simulink model "inverseDynamicsTest"  (Simulink 7.7)
settings: Solver=FixedStepDiscrete  StartTime=0.0  StopTime=1000  FixedStep=0.01  RelTol=1e-3
libraries: WBCLibrary x7, utility x1
settings Model: Creator=iron  LastModifiedBy=iron

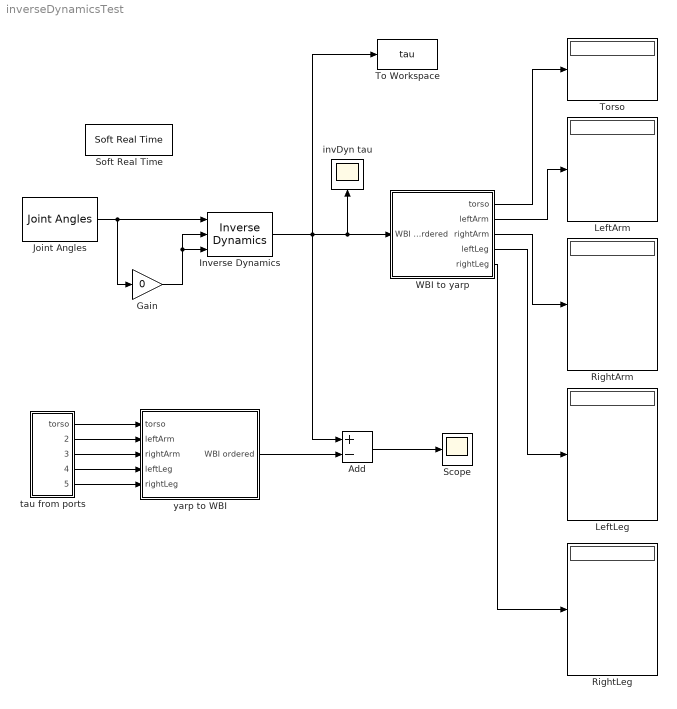
== system inverseDynamicsTest ==
  Add : Sum  Inputs=+-
  Gain : Gain  Gain=0
  Inverse Dynamics : WBCLibrary/wholeBodyModel/Dynamics/Inverse Dynamics  SystemSampleTime=-1  robotName=robotName  localName=localName
  Joint Angles : WBCLibrary/wholeBodyStates/Joint Angles  SystemSampleTime=-1  robotName=robotName  localName=localName
  LeftArm : Display
  LeftLeg : Display
  RightArm : Display
  RightLeg : Display
  Scope : Scope
      settings: YMin=-1.75  YMax=2.5
  Soft Real Time : utility/Soft Real Time  x=0.01
  To Workspace : ToWorkspace  VariableName=tau  SampleTime=-1  SaveFormat=Structure
  Torso : Display
  WBI to yarp : Subsystem
  invDyn tau : Scope
      settings: YMax=1.5
  tau from ports : Subsystem
  yarp to WBI : Subsystem
  wires:
  Joint Angles/1 -> Gain/1, Inverse Dynamics/1
  Gain/1 -> Inverse Dynamics/2, Inverse Dynamics/3
  Inverse Dynamics/1 -> To Workspace/1, Add/1, WBI to yarp/1(WBI ordered), invDyn tau/1
  Add/1 -> Scope/1
  yarp to WBI/1(WBI ordered) -> Add/2
  WBI to yarp/1(torso) -> Torso/1
  WBI to yarp/2(leftArm) -> LeftArm/1
  WBI to yarp/3(rightArm) -> RightArm/1
  WBI to yarp/4(leftLeg) -> LeftLeg/1
  WBI to yarp/5(rightLeg) -> RightLeg/1
  tau from ports/2(leftArm) -> yarp to WBI/2(leftArm)
  tau from ports/1(torso) -> yarp to WBI/1(torso)
  tau from ports/5(rightLeg) -> yarp to WBI/5(rightLeg)
  tau from ports/3(rightArm) -> yarp to WBI/3(rightArm)
  tau from ports/4(leftLeg) -> yarp to WBI/4(leftLeg)

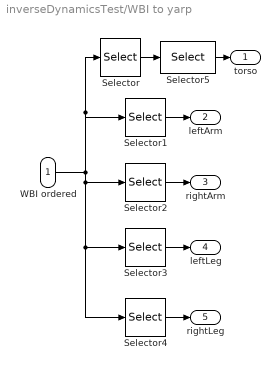
== system inverseDynamicsTest/WBI to yarp ==
  WBI ordered : Inport
  Selector : Selector  InputPortWidth=25  IndexOptions=Index vector (dialog)  Indices=[1 2 3]  OutputSizes=1
  Selector1 : Selector  InputPortWidth=25  IndexOptions=Index vector (dialog)  Indices=[4 5 6 7 8]  OutputSizes=1
  Selector2 : Selector  InputPortWidth=25  IndexOptions=Index vector (dialog)  Indices=[9 10 11 12 13]  OutputSizes=1
  Selector3 : Selector  InputPortWidth=25  IndexOptions=Index vector (dialog)  Indices=[14 15 16 17 18 19]  OutputSizes=1
  Selector4 : Selector  InputPortWidth=25  IndexOptions=Index vector (dialog)  Indices=[20 21 22 23 24 25]  OutputSizes=1
  Selector5 : Selector  InputPortWidth=3  IndexOptions=Index vector (dialog)  Indices=[3 2 1]  OutputSizes=1
  torso : Outport
  leftArm : Outport  Port=2
  rightArm : Outport  Port=3
  leftLeg : Outport  Port=4
  rightLeg : Outport  Port=5
  wires:
  Selector1/1 -> leftArm/1
  Selector2/1 -> rightArm/1
  Selector3/1 -> leftLeg/1
  Selector4/1 -> rightLeg/1
  WBI ordered/1 -> Selector/1, Selector1/1, Selector2/1, Selector4/1, Selector3/1
  Selector/1 -> Selector5/1
  Selector5/1 -> torso/1

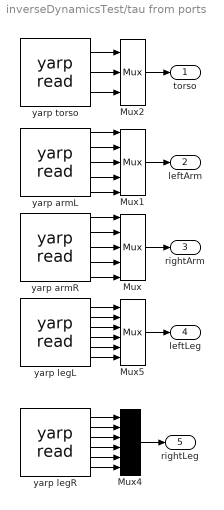
== system inverseDynamicsTest/tau from ports ==
  Mux : Mux  Inputs=5
  Mux1 : Mux  Inputs=5
  Mux2 : Mux  Inputs=3
  Mux4 : Mux  Inputs=6
  Mux5 : Mux  Inputs=6
  yarp armL : WBCLibrary/Utilities/yarp read  from='/icubGazeboSim/left_arm/analog:o/torques'  to='/tmp2:i'  num=5
  yarp armR : WBCLibrary/Utilities/yarp read  from='/icubGazeboSim/right_arm/analog:o/torques'  to='/tmp3:i'  num=5
  yarp legL : WBCLibrary/Utilities/yarp read  from='/icubGazeboSim/left_leg/analog:o/torques'  to='/tmp4:i'  num=6
  yarp legR : WBCLibrary/Utilities/yarp read  from='/icubGazeboSim/right_leg/analog:o/torques'  to='/tmp5:i'  num=6
  yarp torso : WBCLibrary/Utilities/yarp read  from='/icubGazeboSim/torso/analog:o/torques'  to='/tmp1:i'  num=3
  torso : Outport
  leftArm : Outport  Port=2
  rightArm : Outport  Port=3
  leftLeg : Outport  Port=4
  rightLeg : Outport  Port=5
  wires:
  yarp armR/1 -> Mux/1
  yarp armR/2 -> Mux/2
  yarp armR/3 -> Mux/3
  yarp armR/4 -> Mux/4
  yarp armR/5 -> Mux/5
  yarp armL/1 -> Mux1/1
  yarp armL/2 -> Mux1/2
  yarp armL/3 -> Mux1/3
  yarp armL/4 -> Mux1/4
  yarp armL/5 -> Mux1/5
  yarp torso/1 -> Mux2/1
  yarp torso/2 -> Mux2/2
  yarp torso/3 -> Mux2/3
  yarp legL/1 -> Mux5/1
  yarp legL/2 -> Mux5/2
  yarp legL/3 -> Mux5/3
  yarp legL/4 -> Mux5/4
  yarp legL/5 -> Mux5/5
  yarp legL/6 -> Mux5/6
  yarp legR/1 -> Mux4/1
  yarp legR/2 -> Mux4/2
  yarp legR/3 -> Mux4/3
  yarp legR/4 -> Mux4/4
  yarp legR/5 -> Mux4/5
  yarp legR/6 -> Mux4/6
  Mux2/1 -> torso/1
  Mux1/1 -> leftArm/1
  Mux/1 -> rightArm/1
  Mux5/1 -> leftLeg/1
  Mux4/1 -> rightLeg/1

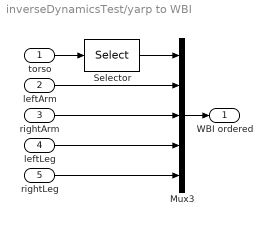
== system inverseDynamicsTest/yarp to WBI ==
  torso : Inport
  leftArm : Inport  Port=2
  rightArm : Inport  Port=3
  leftLeg : Inport  Port=4
  rightLeg : Inport  Port=5
  Mux3 : Mux  Inputs=5
  Selector : Selector  InputPortWidth=3  IndexOptions=Index vector (dialog)  Indices=[3 2 1]  OutputSizes=1
  WBI ordered : Outport
  wires:
  Selector/1 -> Mux3/1
  torso/1 -> Selector/1
  leftArm/1 -> Mux3/2
  rightArm/1 -> Mux3/3
  Mux3/1 -> WBI ordered/1
  leftLeg/1 -> Mux3/4
  rightLeg/1 -> Mux3/5
